simulink library "UoA_3D_LRd_2008"  (R2014b)
settings: Solver=ode45  StartTime=0.0  StopTime=10.0  RelTol=1e-3
libraries: simulink_extras x2, simulink x2
settings Model: Creator=eyip002-admin  LastModifiedBy=nall426

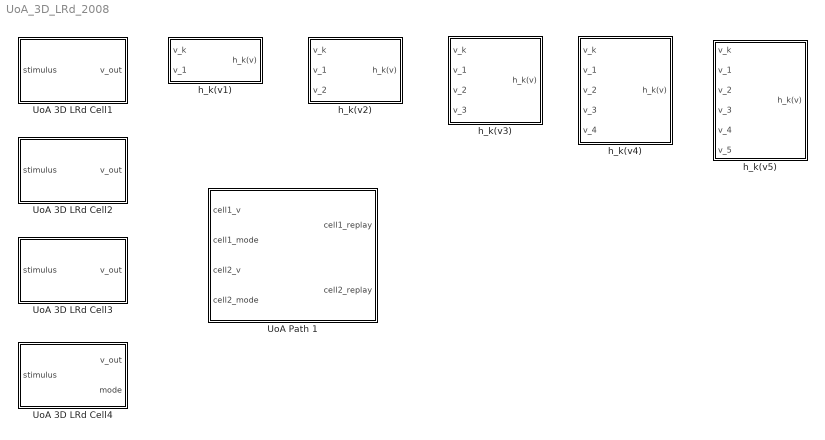
== system UoA_3D_LRd_2008 ==
  UoA 3D LRd Cell1 : Subsystem  mask{V_T=44.5, V_R=30, V_O_max=131.1, alpha0_x=-0.0087, alpha1_x=-0.0236, alpha2_x=-0.0069, alpha3_x=-0.0332, alpha0_y=-0.1909, alpha1_y=-0.0455, alpha2_y=0.0759, alpha3_y=0.0280, alpha0_z=-0.1904, alpha1_z=-0.0129, alpha2_z=6.8265, alpha3_z=0.0020, v_n_R_max=5e-9, v_n_R_min=3.04e-9, i_st_x=0, i_st_y=0, i_st_z=0, i_st_gx=0.7772, i_st_gy=0.0589, i_st_gz=0.2766}
      mask prompts: V_T "V_T (stimulation)"; V_R "V_R (resting)"; V_O_max "V_O_max (overshoot)"; v_n_R_max "v_n_R_max (Maximum rate)"; v_n_R_min "v_n_R_min (To correct transition error)"; i_st_x "i_st_x (x dimension)"; i_st_y "i_st_y (y dimension)"; i_st_z "i_st_z (z dimension)"
      mask DialogControl DescTextVar Prompt: Parameters for UoA 3D Luo-Rudy cardiac cell. Based on Stony Brook's 2008 3D HA LRd model with modifications.
      mask Display:
      | disp('Isolated_1\n(2008)')
      | port_label('input', 1, 'stim')
      | port_label('output', 1, 'v_k')
  UoA 3D LRd Cell2 : Subsystem  mask{V_T=44.5, V_R=30, V_O_max=131.1, alpha0_x=-0.0087, alpha1_x=-0.0236, alpha2_x=-0.0069, alpha3_x=-0.0332, alpha0_y=-0.1909, alpha1_y=-0.0455, alpha2_y=0.0759, alpha3_y=0.0280, alpha0_z=-0.1904, alpha1_z=-0.0129, alpha2_z=6.8265, alpha3_z=0.0020, v_n_R_max=5e-9, v_n_R_min=3.04e-9, i_st_x=0, i_st_y=0, i_st_z=0, i_st_gx=0.7772, i_st_gy=0.0589, i_st_gz=0.2766}
      mask prompts: V_T "V_T (stimulation)"; V_R "V_R (resting)"; V_O_max "V_O_max (overshoot)"; v_n_R_max "v_n_R_max (Maximum rate)"; v_n_R_min "v_n_R_min (To correct transition error)"; i_st_x "i_st_x (x dimension)"; i_st_y "i_st_y (y dimension)"; i_st_z "i_st_z (z dimension)"
      mask DialogControl DescTextVar Prompt: Parameters for UoA 3D Luo-Rudy cardiac cell. Based on Stony Brook's 2008 3D HA LRd model with modifications.
      mask Display:
      | disp('Isolated_2\n(2008)')
      | port_label('input', 1, 'stim')
      | port_label('output', 1, 'v_k')
  UoA 3D LRd Cell3 : Subsystem  mask{V_T=44.5, V_R=30, V_O_max=131.1, alpha0_x=-0.0087, alpha1_x=-0.0236, alpha2_x=-0.0069, alpha3_x=-0.0332, alpha0_y=-0.1909, alpha1_y=-0.0455, alpha2_y=0.0759, alpha3_y=0.0280, alpha0_z=-0.1904, alpha1_z=-0.0129, alpha2_z=6.8265, alpha3_z=0.0020, v_n_R_max=0.04, i_st_gx=0.7772, i_st_gy=0.0589, i_st_gz=0.2766}
      mask prompts: V_T "V_T (stimulation)"; V_R "V_R (resting)"; V_O_max "V_O_max (overshoot)"; v_n_R_max "v_n_R_max (Maximum rate)"
      mask DialogControl DescTextVar Prompt: Parameters for UoA 3D Luo-Rudy cardiac cell. Based on Stony Brook's 2008 3D HA LRd model with modifications.
      mask DialogControl Container10 Prompt: Stimulus current as a proportion of incoming voltages
      mask Display:
      | disp('Isolated_3\n(2008)')
      | port_label('input', 1, 'stim')
      | port_label('output', 1, 'v_k')
  UoA 3D LRd Cell4 : Subsystem  mask{V_T=44.5, V_R=30, V_O_max=131.1, alpha0_x=-0.0087, alpha1_x=-0.0236, alpha2_x=-0.0069, alpha3_x=-0.0332, alpha0_y=-0.1909, alpha1_y=-0.0455, alpha2_y=0.0759, alpha3_y=0.0280, alpha0_z=-0.1904, alpha1_z=-0.0129, alpha2_z=6.8265, alpha3_z=0.0020, v_n_R_max=0.04, i_st_gx=0.7772, i_st_gy=0.0589, i_st_gz=0.2766}
      mask prompts: V_T "V_T (stimulation)"; V_R "V_R (resting)"; V_O_max "V_O_max (overshoot)"; v_n_R_max "v_n_R_max (Maximum rate)"
      mask DialogControl DescTextVar Prompt: Parameters for UoA 3D Luo-Rudy cardiac cell. Based on Stony Brook's 3D HA LRd model with modifications.
      mask DialogControl Container10 Prompt: Stimulus current as a proportion of incoming voltages
      mask Display:
      | disp('Isolated_4\n(2008)')
      | port_label('input', 1, 'stim')
      | port_label('output', 1, 'v_k')
      | port_label('output', 2, 'mode')
  UoA Path 1 : Subsystem  mask{cell1_conduction_time=1, cell2_conduction_time=1, cell1_charge_time=1, cell2_charge_time=1}
      mask prompts: cell1_conduction_time "Cell 1 to cell 2"; cell2_conduction_time "Cell 2 to cell 1"; cell1_charge_time "Cell 1"; cell2_charge_time "Cell 2"
      mask DialogControl DescTextVar Prompt: Parameters for the UoA path model. Based on the UPenn path model with modifications.
      mask Display:
      | disp('UoA_1')
      | port_label('input', 1, 'cell1_v')
      | port_label('input', 2, 'cell1_mode')
      | port_label('input', 3, 'cell2_v')
      | port_label('input', 4, 'cell2_mode')
      | port_label('output', 1, 'cell1_replay')
      | port_label('output', 2, 'cell2_replay')
  h_k(v1) : Subsystem  mask{A_m=10*10, C_m=1/(10*10), G_1=10*10, s_1=1/10, d_1=10}
      mask prompts: A_m "A_m (Cell surface area to cell volume)"; C_m "C_m (Specific membrane capacitance)"
      mask DialogControl DescTextVar Prompt: University of Auckland's voltage aggregation function, h(v).
      mask Display:
      | disp('UoA_1')
      | port_label('input', 1, 'v_k')
      | port_label('input', 2, 'v_1')
      | port_label('output', 1, 'h_k')
  h_k(v2) : Subsystem  mask{A_m=10*10, C_m=1/(10*10), G_1=10*10, G_2=10*10, s_1=1/10, s_2=1/10, d_1=10, d_2=10}
      mask prompts: A_m "A_m (Cell surface area to cell volume)"; C_m "C_m (Specific membrane capacitance)"
      mask DialogControl DescTextVar Prompt: University of Auckland's voltage aggregation function, h(v).
      mask Display:
      | disp('UoA_1')
      | port_label('input', 1, 'v_k')
      | port_label('input', 2, 'v_1')
      | port_label('input', 3, 'v_2')
      | port_label('output', 1, 'h_k')
  h_k(v3) : Subsystem  mask{A_m=10*10, C_m=1/(10*10), G_1=10*10, G_2=10*10, G_3=10*10, s_1=1/10, s_2=1/10, s_3=1/10, d_1=10, d_2=10, d_3=10}
      mask prompts: A_m "A_m (Cell surface area to cell volume)"; C_m "C_m (Specific membrane capacitance)"
      mask DialogControl DescTextVar Prompt: University of Auckland's voltage aggregation function, h(v).
      mask Display:
      | disp('UoA_1')
      | port_label('input', 1, 'v_k')
      | port_label('input', 2, 'v_1')
      | port_label('input', 3, 'v_2')
      | port_label('input', 4, 'v_3')
      | port_label('output', 1, 'h_k')
  h_k(v4) : Subsystem  mask{A_m=10*10, C_m=1/(10*10), G_1=10*10, G_2=10*10, G_3=10*10, G_4=10*10, s_1=1/10, s_2=1/10, s_3=1/10, s_4=1/10, d_1=10, d_2=10, d_3=10, d_4=10}
      mask prompts: A_m "A_m (Cell surface area to cell volume)"; C_m "C_m (Specific membrane capacitance)"
      mask DialogControl DescTextVar Prompt: University of Auckland's voltage aggregation function, h(v).
      mask Display:
      | disp('UoA_1')
      | port_label('input', 1, 'v_k')
      | port_label('input', 2, 'v_1')
      | port_label('input', 3, 'v_2')
      | port_label('input', 4, 'v_3')
      | port_label('input', 5, 'v_4')
      | port_label('output', 1, 'h_k')
  h_k(v5) : Subsystem  mask{A_m=10*10, C_m=1/(10*10), G_1=10*10, G_2=10*10, G_3=10*10, G_4=10*10, G_5=10*10, s_1=1/10, s_2=1/10, s_3=1/10, s_4=1/10, s_5=1/10, d_1=10, d_2=10, d_3=10, d_4=10, d_5=10}
      mask prompts: A_m "A_m (Cell surface area to cell volume)"; C_m "C_m (Specific membrane capacitance)"
      mask DialogControl DescTextVar Prompt: University of Auckland's voltage aggregation function, h(v).
      mask Display:
      | disp('UoA_1')
      | port_label('input', 1, 'v_k')
      | port_label('input', 2, 'v_1')
      | port_label('input', 3, 'v_2')
      | port_label('input', 4, 'v_3')
      | port_label('input', 5, 'v_4')
      | port_label('input', 6, 'v_5')
      | port_label('output', 1, 'h_k')

== system UoA_3D_LRd_2008/UoA 3D LRd Cell1 ==
  stimulus : Inport
  Modes and Transitions : Stateflow chart  TreatAsAtomicUnit=on
  V_O_max : Constant  Value=V_O_max
  V_R : Constant  Value=V_R
  V_T : Constant  Value=V_T
  v_(x,y,z) Computation : Subsystem
  v_out : Outport
  wires:
  Modes and Transitions/2(v_n_R) -> v_(x,y,z) Computation/3(v_n_R)
  Modes and Transitions/1(Mode) -> v_(x,y,z) Computation/2(Mode)
  v_(x,y,z) Computation/2(v_x_next) -> Modes and Transitions/5(v_x)
  Modes and Transitions/3(v_x_reset) -> v_(x,y,z) Computation/4(v_x_reset)
  Modes and Transitions/6(reset) -> v_(x,y,z) Computation/7(reset)
  v_(x,y,z) Computation/3(v_y_next) -> Modes and Transitions/6(v_y)
  v_(x,y,z) Computation/4(v_z_next) -> Modes and Transitions/7(v_z)
  Modes and Transitions/4(v_y_reset) -> v_(x,y,z) Computation/5(v_y_reset)
  Modes and Transitions/5(v_z_reset) -> v_(x,y,z) Computation/6(v_z_reset)
  stimulus/1 -> v_(x,y,z) Computation/1(g(v)), Modes and Transitions/1(stimulus)
  v_(x,y,z) Computation/1(v_out) -> v_out/1
  V_T/1 -> Modes and Transitions/2(V_T)
  V_R/1 -> Modes and Transitions/3(V_R)
  V_O_max/1 -> Modes and Transitions/4(V_O_max)

== system UoA_3D_LRd_2008/UoA 3D LRd Cell2 ==
  stimulus : Inport
  Modes and Transitions : Stateflow chart  TreatAsAtomicUnit=on
  V_O_max : Constant  Value=V_O_max
  V_R : Constant  Value=V_R
  V_T : Constant  Value=V_T
  v_(x,y,z) Computation : Subsystem
  v_out : Outport
  wires:
  Modes and Transitions/2(v_n_R) -> v_(x,y,z) Computation/3(v_n_R)
  Modes and Transitions/1(Mode) -> v_(x,y,z) Computation/2(Mode)
  v_(x,y,z) Computation/2(v_x_next) -> Modes and Transitions/5(v_x)
  Modes and Transitions/3(v_x_reset) -> v_(x,y,z) Computation/4(v_x_reset)
  Modes and Transitions/6(reset) -> v_(x,y,z) Computation/7(reset)
  v_(x,y,z) Computation/3(v_y_next) -> Modes and Transitions/6(v_y)
  v_(x,y,z) Computation/4(v_z_next) -> Modes and Transitions/7(v_z)
  Modes and Transitions/4(v_y_reset) -> v_(x,y,z) Computation/5(v_y_reset)
  Modes and Transitions/5(v_z_reset) -> v_(x,y,z) Computation/6(v_z_reset)
  stimulus/1 -> v_(x,y,z) Computation/1(g(v)), Modes and Transitions/1(stimulus)
  v_(x,y,z) Computation/1(v_out) -> v_out/1
  V_T/1 -> Modes and Transitions/2(V_T)
  V_R/1 -> Modes and Transitions/3(V_R)
  V_O_max/1 -> Modes and Transitions/4(V_O_max)

== system UoA_3D_LRd_2008/UoA 3D LRd Cell3 ==
  stimulus : Inport
  Modes and Transitions : Stateflow chart  TreatAsAtomicUnit=on
  V_O_max : Constant  Value=V_O_max
  V_R : Constant  Value=V_R
  V_T : Constant  Value=V_T
  v_(x,y,z) Computation : Subsystem
  v_out : Outport
  wires:
  Modes and Transitions/2(v_n_R) -> v_(x,y,z) Computation/3(v_n_R)
  Modes and Transitions/1(Mode) -> v_(x,y,z) Computation/2(Mode)
  v_(x,y,z) Computation/2(v_x_next) -> Modes and Transitions/5(v_x)
  Modes and Transitions/3(v_x_reset) -> v_(x,y,z) Computation/4(v_x_reset)
  Modes and Transitions/6(reset) -> v_(x,y,z) Computation/7(reset)
  v_(x,y,z) Computation/3(v_y_next) -> Modes and Transitions/6(v_y)
  v_(x,y,z) Computation/4(v_z_next) -> Modes and Transitions/7(v_z)
  Modes and Transitions/4(v_y_reset) -> v_(x,y,z) Computation/5(v_y_reset)
  Modes and Transitions/5(v_z_reset) -> v_(x,y,z) Computation/6(v_z_reset)
  stimulus/1 -> v_(x,y,z) Computation/1(g(v)), Modes and Transitions/1(stimulus)
  v_(x,y,z) Computation/1(v_out) -> v_out/1
  V_T/1 -> Modes and Transitions/2(V_T)
  V_R/1 -> Modes and Transitions/3(V_R)
  V_O_max/1 -> Modes and Transitions/4(V_O_max)

== system UoA_3D_LRd_2008/UoA 3D LRd Cell4 ==
  stimulus : Inport
  Modes and Transitions : Stateflow chart  TreatAsAtomicUnit=on
  V_O_max : Constant  Value=V_O_max
  V_R : Constant  Value=V_R
  V_T : Constant  Value=V_T
  v_(x,y,z) Computation : Subsystem
  v_out : Outport
  mode : Outport  Port=2
  wires:
  V_O_max/1 -> Modes and Transitions/4(V_O_max)
  V_R/1 -> Modes and Transitions/3(V_R)
  V_T/1 -> Modes and Transitions/2(V_T)
  v_(x,y,z) Computation/1(v_out) -> v_out/1
  stimulus/1 -> Modes and Transitions/1(stimulus), v_(x,y,z) Computation/1(g(v))
  Modes and Transitions/5(v_z_reset) -> v_(x,y,z) Computation/6(v_z_reset)
  Modes and Transitions/4(v_y_reset) -> v_(x,y,z) Computation/5(v_y_reset)
  v_(x,y,z) Computation/4(v_z_next) -> Modes and Transitions/7(v_z)
  v_(x,y,z) Computation/3(v_y_next) -> Modes and Transitions/6(v_y)
  Modes and Transitions/6(reset) -> v_(x,y,z) Computation/7(reset)
  Modes and Transitions/3(v_x_reset) -> v_(x,y,z) Computation/4(v_x_reset)
  v_(x,y,z) Computation/2(v_x_next) -> Modes and Transitions/5(v_x)
  Modes and Transitions/1(Mode) -> mode/1, v_(x,y,z) Computation/2(Mode)
  Modes and Transitions/2(v_n_R) -> v_(x,y,z) Computation/3(v_n_R)

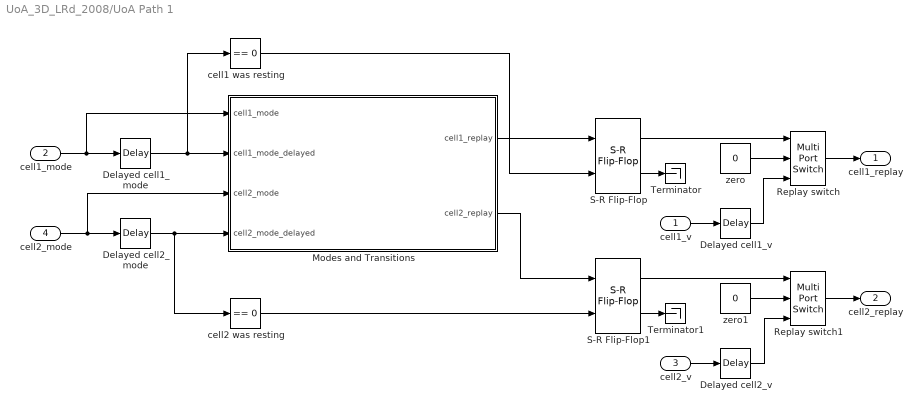
== system UoA_3D_LRd_2008/UoA Path 1 ==
  cell1_v : Inport
  cell1_mode : Inport  Port=2
  cell2_v : Inport  Port=3
  cell2_mode : Inport  Port=4
  Delayed cell1_mode : TransportDelay  DelayTime=cell1_conduction_time  BufferSize=200704
  Delayed cell1_v : TransportDelay  DelayTime=cell1_conduction_time  BufferSize=200704
  Delayed cell2_mode : TransportDelay  DelayTime=cell2_conduction_time  BufferSize=200704
  Delayed cell2_v : TransportDelay  DelayTime=cell2_conduction_time  BufferSize=200704
  Modes and Transitions : Stateflow chart  TreatAsAtomicUnit=on
  Replay switch : MultiPortSwitch  DataPortOrder=Zero-based contiguous  Inputs=2
  Replay switch1 : MultiPortSwitch  DataPortOrder=Zero-based contiguous  Inputs=2
  S-R Flip-Flop : simulink_extras/Flip Flops/S-R Flip-Flop  initial_condition=0
  S-R Flip-Flop1 : simulink_extras/Flip Flops/S-R Flip-Flop  initial_condition=0
  Terminator : Terminator
  Terminator1 : Terminator
  cell1 was resting : simulink/Logic and Bit Operations/Compare To Constant  relop===  const=0  OutDataTypeStr=boolean
  cell2 was resting : simulink/Logic and Bit Operations/Compare To Constant  relop===  const=0  OutDataTypeStr=boolean
  zero : Constant  Value=0
  zero1 : Constant  Value=0
  cell1_replay : Outport
  cell2_replay : Outport  Port=2
  wires:
  cell2_mode/1 -> Modes and Transitions/3(cell2_mode), Delayed cell2_mode/1
  cell1_mode/1 -> Modes and Transitions/1(cell1_mode), Delayed cell1_mode/1
  Replay switch/1 -> cell1_replay/1
  Replay switch1/1 -> cell2_replay/1
  zero/1 -> Replay switch/2
  zero1/1 -> Replay switch1/2
  cell2_v/1 -> Delayed cell2_v/1
  cell1_v/1 -> Delayed cell1_v/1
  Delayed cell2_v/1 -> Replay switch1/3
  Delayed cell1_v/1 -> Replay switch/3
  Delayed cell2_mode/1 -> Modes and Transitions/4(cell2_mode_delayed), cell2 was resting/1
  Delayed cell1_mode/1 -> cell1 was resting/1, Modes and Transitions/2(cell1_mode_delayed)
  S-R Flip-Flop1/1 -> Replay switch1/1
  S-R Flip-Flop1/2 -> Terminator1/1
  S-R Flip-Flop/2 -> Terminator/1
  S-R Flip-Flop/1 -> Replay switch/1
  Modes and Transitions/2(cell2_replay) -> S-R Flip-Flop1/1
  Modes and Transitions/1(cell1_replay) -> S-R Flip-Flop/1
  cell1 was resting/1 -> S-R Flip-Flop/2
  cell2 was resting/1 -> S-R Flip-Flop1/2

== system UoA_3D_LRd_2008/h_k(v1) ==
  v_k : Inport
  v_1 : Inport  Port=2
  Diffusion_1 : Constant  Value=(G_1*s_1)/(A_m*C_m*d_1)
  Product : Product
  Subtract : Sum  Inputs=+-
  h_k(v) : Outport
  wires:
  Product/1 -> h_k(v)/1
  v_k/1 -> Subtract/2
  v_1/1 -> Subtract/1
  Subtract/1 -> Product/2
  Diffusion_1/1 -> Product/1

== system UoA_3D_LRd_2008/h_k(v2) ==
  v_k : Inport
  v_1 : Inport  Port=2
  v_2 : Inport  Port=3
  Diffusion_1 : Constant  Value=(G_1*s_1)/(A_m*C_m*d_1)
  Diffusion_2 : Constant  Value=(G_2*s_2)/(A_m*C_m*d_2)
  Product : Product
  Product1 : Product
  Subtract : Sum  Inputs=+-
  Subtract1 : Sum  Inputs=+-
  Sum : Sum
  h_k(v) : Outport
  wires:
  Sum/1 -> h_k(v)/1
  v_k/1 -> Subtract/2, Subtract1/2
  v_1/1 -> Subtract/1
  Subtract/1 -> Product/2
  Diffusion_1/1 -> Product/1
  Product/1 -> Sum/1
  v_2/1 -> Subtract1/1
  Subtract1/1 -> Product1/2
  Diffusion_2/1 -> Product1/1
  Product1/1 -> Sum/2

== system UoA_3D_LRd_2008/h_k(v3) ==
  v_k : Inport
  v_1 : Inport  Port=2
  v_2 : Inport  Port=3
  v_3 : Inport  Port=4
  Diffusion_1 : Constant  Value=(G_1*s_1)/(A_m*C_m*d_1)
  Diffusion_2 : Constant  Value=(G_2*s_2)/(A_m*C_m*d_2)
  Diffusion_3 : Constant  Value=(G_3*s_3)/(A_m*C_m*d_3)
  Product : Product
  Product1 : Product
  Product2 : Product
  Subtract : Sum  Inputs=+-
  Subtract1 : Sum  Inputs=+-
  Subtract2 : Sum  Inputs=+-
  Sum : Sum  Inputs=+++
  h_k(v) : Outport
  wires:
  Sum/1 -> h_k(v)/1
  v_1/1 -> Subtract/1
  Subtract/1 -> Product/2
  Diffusion_1/1 -> Product/1
  Product/1 -> Sum/1
  v_2/1 -> Subtract1/1
  Subtract1/1 -> Product1/2
  Diffusion_2/1 -> Product1/1
  Product1/1 -> Sum/2
  v_k/1 -> Subtract/2, Subtract1/2, Subtract2/2
  v_3/1 -> Subtract2/1
  Subtract2/1 -> Product2/2
  Diffusion_3/1 -> Product2/1
  Product2/1 -> Sum/3

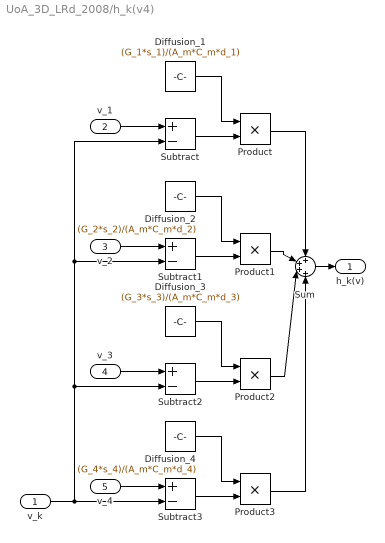
== system UoA_3D_LRd_2008/h_k(v4) ==
  v_k : Inport
  v_1 : Inport  Port=2
  v_2 : Inport  Port=3
  v_3 : Inport  Port=4
  v_4 : Inport  Port=5
  Diffusion_1 : Constant  Value=(G_1*s_1)/(A_m*C_m*d_1)
  Diffusion_2 : Constant  Value=(G_2*s_2)/(A_m*C_m*d_2)
  Diffusion_3 : Constant  Value=(G_3*s_3)/(A_m*C_m*d_3)
  Diffusion_4 : Constant  Value=(G_4*s_4)/(A_m*C_m*d_4)
  Product{,1..3} (4 alike) : Product
  Subtract{,1..3} (4 alike) : Sum  Inputs=+-
  Sum : Sum  Inputs=++++
  h_k(v) : Outport
  wires:
  Sum/1 -> h_k(v)/1
  v_1/1 -> Subtract/1
  Subtract/1 -> Product/2
  Diffusion_1/1 -> Product/1
  Product/1 -> Sum/1
  v_2/1 -> Subtract1/1
  Subtract1/1 -> Product1/2
  Diffusion_2/1 -> Product1/1
  Product1/1 -> Sum/2
  v_3/1 -> Subtract2/1
  Subtract2/1 -> Product2/2
  Diffusion_3/1 -> Product2/1
  Product2/1 -> Sum/3
  v_k/1 -> Subtract/2, Subtract1/2, Subtract2/2, Subtract3/2
  v_4/1 -> Subtract3/1
  Subtract3/1 -> Product3/2
  Diffusion_4/1 -> Product3/1
  Product3/1 -> Sum/4

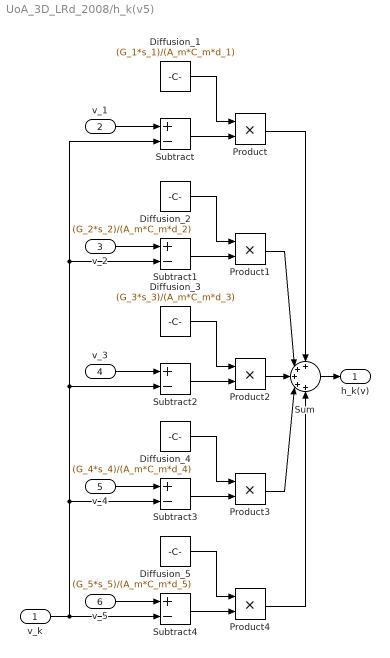
== system UoA_3D_LRd_2008/h_k(v5) ==
  v_k : Inport
  v_1 : Inport  Port=2
  v_2 : Inport  Port=3
  v_3 : Inport  Port=4
  v_4 : Inport  Port=5
  v_5 : Inport  Port=6
  Diffusion_1 : Constant  Value=(G_1*s_1)/(A_m*C_m*d_1)
  Diffusion_2 : Constant  Value=(G_2*s_2)/(A_m*C_m*d_2)
  Diffusion_3 : Constant  Value=(G_3*s_3)/(A_m*C_m*d_3)
  Diffusion_4 : Constant  Value=(G_4*s_4)/(A_m*C_m*d_4)
  Diffusion_5 : Constant  Value=(G_5*s_5)/(A_m*C_m*d_5)
  Product{,1..4} (5 alike) : Product
  Subtract{,1..4} (5 alike) : Sum  Inputs=+-
  Sum : Sum  Inputs=+++++
  h_k(v) : Outport
  wires:
  Sum/1 -> h_k(v)/1
  v_1/1 -> Subtract/1
  Subtract/1 -> Product/2
  Diffusion_1/1 -> Product/1
  Product/1 -> Sum/1
  v_2/1 -> Subtract1/1
  Subtract1/1 -> Product1/2
  Diffusion_2/1 -> Product1/1
  Product1/1 -> Sum/2
  v_3/1 -> Subtract2/1
  Subtract2/1 -> Product2/2
  Diffusion_3/1 -> Product2/1
  Product2/1 -> Sum/3
  v_4/1 -> Subtract3/1
  Subtract3/1 -> Product3/2
  Diffusion_4/1 -> Product3/1
  Product3/1 -> Sum/4
  v_k/1 -> Subtract4/2, Subtract/2, Subtract1/2, Subtract2/2, Subtract3/2
  v_5/1 -> Subtract4/1
  Subtract4/1 -> Product4/2
  Diffusion_5/1 -> Product4/1
  Product4/1 -> Sum/5

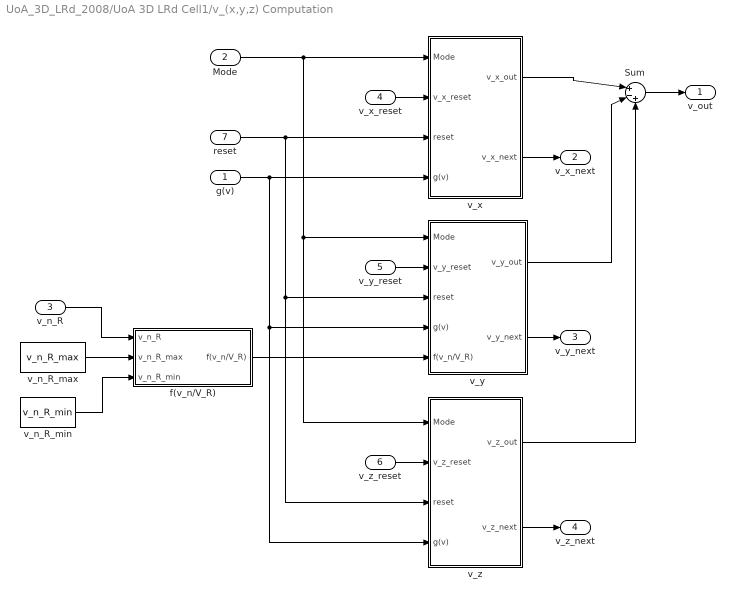
== system UoA_3D_LRd_2008/UoA 3D LRd Cell1/v_(x,y,z) Computation ==
  g(v) : Inport
  Mode : Inport  Port=2
  v_n_R : Inport  Port=3
  v_x_reset : Inport  Port=4
  v_y_reset : Inport  Port=5
  v_z_reset : Inport  Port=6
  reset : Inport  Port=7
  Sum : Sum  Inputs=|+-+
  f(v_n/V_R) : Subsystem
  v_n_R_max : Constant  Value=v_n_R_max
  v_n_R_min : Constant  Value=v_n_R_min
  v_x : Subsystem
  v_y : Subsystem
  v_z : Subsystem
  v_out : Outport
  v_x_next : Outport  Port=2
  v_y_next : Outport  Port=3
  v_z_next : Outport  Port=4
  wires:
  v_x_reset/1 -> v_x/2(v_x_reset)
  v_x/2(v_x_next) -> v_x_next/1
  v_y/2(v_y_next) -> v_y_next/1
  Mode/1 -> v_z/1(Mode), v_y/1(Mode), v_x/1(Mode)
  v_z/2(v_z_next) -> v_z_next/1
  Sum/1 -> v_out/1
  v_x/1(v_x_out) -> Sum/1
  v_y/1(v_y_out) -> Sum/2
  v_z/1(v_z_out) -> Sum/3
  v_y_reset/1 -> v_y/2(v_y_reset)
  v_z_reset/1 -> v_z/2(v_z_reset)
  g(v)/1 -> v_x/4(g(v)), v_z/4(g(v)), v_y/4(g(v))
  reset/1 -> v_z/3(reset), v_y/3(reset), v_x/3(reset)
  v_n_R_max/1 -> f(v_n/V_R)/2(v_n_R_max)
  v_n_R/1 -> f(v_n/V_R)/1(v_n_R)
  f(v_n/V_R)/1(f(v_n/V_R)) -> v_y/5(f(v_n/V_R))
  v_n_R_min/1 -> f(v_n/V_R)/3(v_n_R_min)

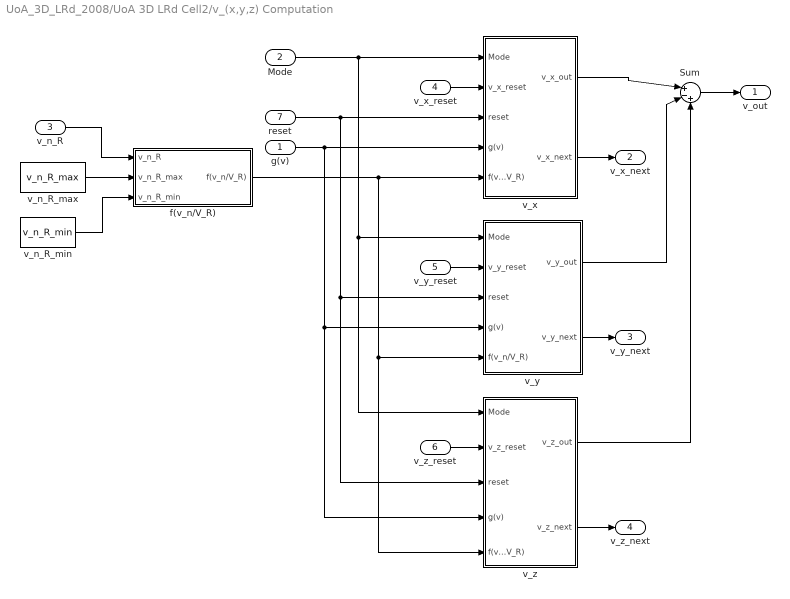
== system UoA_3D_LRd_2008/UoA 3D LRd Cell2/v_(x,y,z) Computation ==
  g(v) : Inport
  Mode : Inport  Port=2
  v_n_R : Inport  Port=3
  v_x_reset : Inport  Port=4
  v_y_reset : Inport  Port=5
  v_z_reset : Inport  Port=6
  reset : Inport  Port=7
  Sum : Sum  Inputs=|+-+
  f(v_n/V_R) : Subsystem
  v_n_R_max : Constant  Value=v_n_R_max
  v_n_R_min : Constant  Value=v_n_R_min
  v_x : Subsystem
  v_y : Subsystem
  v_z : Subsystem
  v_out : Outport
  v_x_next : Outport  Port=2
  v_y_next : Outport  Port=3
  v_z_next : Outport  Port=4
  wires:
  v_x_reset/1 -> v_x/2(v_x_reset)
  v_x/2(v_x_next) -> v_x_next/1
  v_y/2(v_y_next) -> v_y_next/1
  Mode/1 -> v_z/1(Mode), v_y/1(Mode), v_x/1(Mode)
  v_z/2(v_z_next) -> v_z_next/1
  Sum/1 -> v_out/1
  v_x/1(v_x_out) -> Sum/1
  v_y/1(v_y_out) -> Sum/2
  v_z/1(v_z_out) -> Sum/3
  v_y_reset/1 -> v_y/2(v_y_reset)
  v_z_reset/1 -> v_z/2(v_z_reset)
  g(v)/1 -> v_z/4(g(v)), v_y/4(g(v)), v_x/4(g(v))
  reset/1 -> v_z/3(reset), v_y/3(reset), v_x/3(reset)
  v_n_R_max/1 -> f(v_n/V_R)/2(v_n_R_max)
  v_n_R/1 -> f(v_n/V_R)/1(v_n_R)
  f(v_n/V_R)/1(f(v_n/V_R)) -> v_z/5(f(v_n/V_R)), v_y/5(f(v_n/V_R)), v_x/5(f(v_n/V_R))
  v_n_R_min/1 -> f(v_n/V_R)/3(v_n_R_min)

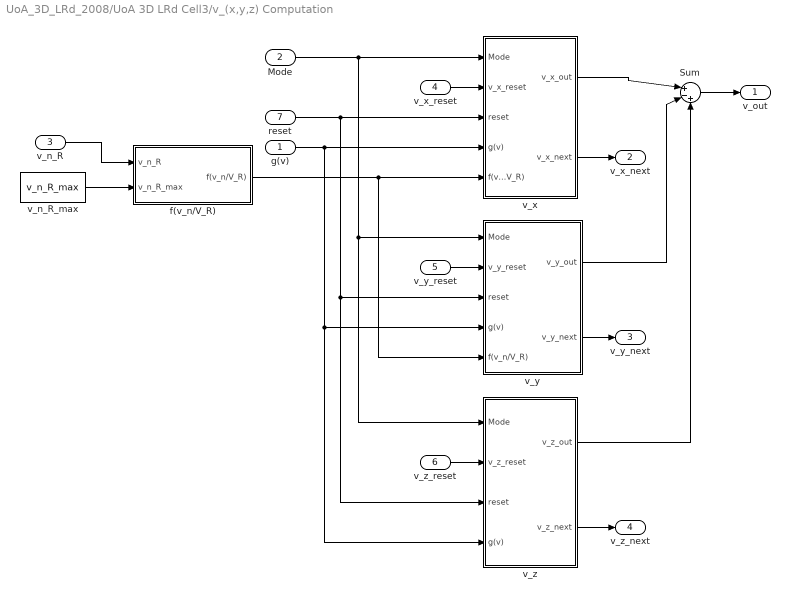
== system UoA_3D_LRd_2008/UoA 3D LRd Cell3/v_(x,y,z) Computation ==
  g(v) : Inport
  Mode : Inport  Port=2
  v_n_R : Inport  Port=3
  v_x_reset : Inport  Port=4
  v_y_reset : Inport  Port=5
  v_z_reset : Inport  Port=6
  reset : Inport  Port=7
  Sum : Sum  Inputs=|+-+
  f(v_n/V_R) : Subsystem
  v_n_R_max : Constant  Value=v_n_R_max
  v_x : Subsystem
  v_y : Subsystem
  v_z : Subsystem
  v_out : Outport
  v_x_next : Outport  Port=2
  v_y_next : Outport  Port=3
  v_z_next : Outport  Port=4
  wires:
  v_x_reset/1 -> v_x/2(v_x_reset)
  v_x/2(v_x_next) -> v_x_next/1
  v_y/2(v_y_next) -> v_y_next/1
  Mode/1 -> v_z/1(Mode), v_y/1(Mode), v_x/1(Mode)
  v_z/2(v_z_next) -> v_z_next/1
  Sum/1 -> v_out/1
  v_x/1(v_x_out) -> Sum/1
  v_y/1(v_y_out) -> Sum/2
  v_z/1(v_z_out) -> Sum/3
  v_y_reset/1 -> v_y/2(v_y_reset)
  v_z_reset/1 -> v_z/2(v_z_reset)
  g(v)/1 -> v_z/4(g(v)), v_y/4(g(v)), v_x/4(g(v))
  reset/1 -> v_z/3(reset), v_y/3(reset), v_x/3(reset)
  v_n_R_max/1 -> f(v_n/V_R)/2(v_n_R_max)
  v_n_R/1 -> f(v_n/V_R)/1(v_n_R)
  f(v_n/V_R)/1(f(v_n/V_R)) -> v_y/5(f(v_n/V_R)), v_x/5(f(v_n/V_R))

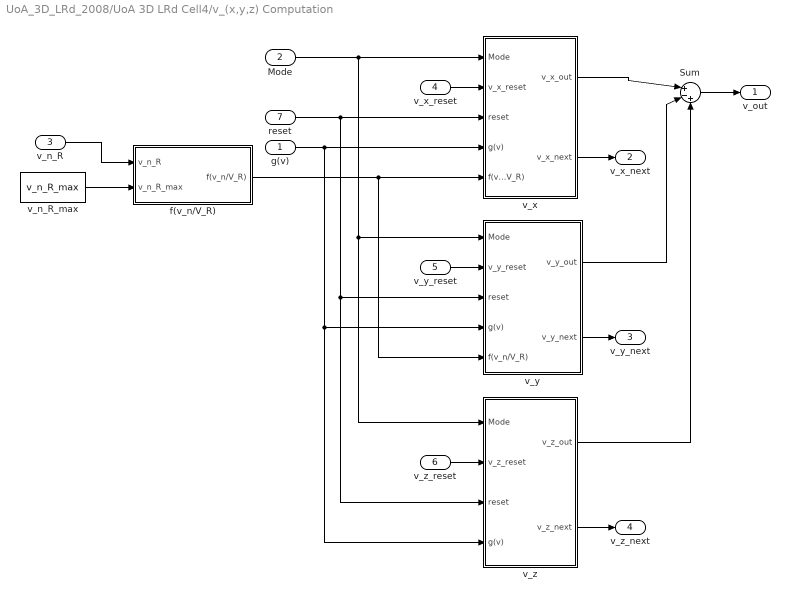
== system UoA_3D_LRd_2008/UoA 3D LRd Cell4/v_(x,y,z) Computation ==
  g(v) : Inport
  Mode : Inport  Port=2
  v_n_R : Inport  Port=3
  v_x_reset : Inport  Port=4
  v_y_reset : Inport  Port=5
  v_z_reset : Inport  Port=6
  reset : Inport  Port=7
  Sum : Sum  Inputs=|+-+
  f(v_n/V_R) : Subsystem
  v_n_R_max : Constant  Value=v_n_R_max
  v_x : Subsystem
  v_y : Subsystem
  v_z : Subsystem
  v_out : Outport
  v_x_next : Outport  Port=2
  v_y_next : Outport  Port=3
  v_z_next : Outport  Port=4
  wires:
  f(v_n/V_R)/1(f(v_n/V_R)) -> v_x/5(f(v_n/V_R)), v_y/5(f(v_n/V_R))
  v_n_R/1 -> f(v_n/V_R)/1(v_n_R)
  v_n_R_max/1 -> f(v_n/V_R)/2(v_n_R_max)
  reset/1 -> v_x/3(reset), v_y/3(reset), v_z/3(reset)
  g(v)/1 -> v_x/4(g(v)), v_y/4(g(v)), v_z/4(g(v))
  v_z_reset/1 -> v_z/2(v_z_reset)
  v_y_reset/1 -> v_y/2(v_y_reset)
  v_z/1(v_z_out) -> Sum/3
  v_y/1(v_y_out) -> Sum/2
  v_x/1(v_x_out) -> Sum/1
  Sum/1 -> v_out/1
  Mode/1 -> v_x/1(Mode), v_y/1(Mode), v_z/1(Mode)
  v_x_reset/1 -> v_x/2(v_x_reset)
  v_z/2(v_z_next) -> v_z_next/1
  v_y/2(v_y_next) -> v_y_next/1
  v_x/2(v_x_next) -> v_x_next/1

== system UoA_3D_LRd_2008/UoA 3D LRd Cell1/v_(x,y,z) Computation/f(v_n//V_R) ==
  v_n_R : Inport
  v_n_R_max : Inport  Port=2
  v_n_R_min : Inport  Port=3
  -10.99 : Gain  Gain=-10.99
  0.29 : Gain  Gain=0.29
  0.70 : Gain  Gain=0.70
  62.89 : Gain  Gain=62.89
  Subtract : Sum  Inputs=-+
  Subtract1 : Sum  Inputs=+-
  Sum3 : Sum  Inputs=|++
  Switch : Switch  Criteria=u2 > Threshold
  Switch1 : Switch  Criteria=u2 > Threshold
  Zero : Constant  Value=0
  exp : Math  SaturateOnIntegerOverflow=on
  exp1 : Math  SaturateOnIntegerOverflow=on
  f(v_n/V_R) : Outport
  wires:
  Sum3/1 -> f(v_n/V_R)/1
  v_n_R_max/1 -> Switch/3, Subtract/2
  Switch1/1 -> Switch/1, Subtract/1
  Subtract/1 -> Switch/2
  ? -> Switch1/3, Subtract1/2
  v_n_R_min/1 -> Subtract1/1
  Subtract1/1 -> Switch1/2
  Zero/1 -> Switch1/1
  62.89/1 -> exp/1
  exp/1 -> 0.29/1
  -10.99/1 -> exp1/1
  exp1/1 -> 0.70/1
  0.29/1 -> Sum3/1
  0.70/1 -> Sum3/2
  v_n_R/1 -> 62.89/1, -10.99/1

== system UoA_3D_LRd_2008/UoA 3D LRd Cell1/v_(x,y,z) Computation/v_x ==
  Mode : Inport
  v_x_reset : Inport  Port=2
  reset : Inport  Port=3
  g(v) : Inport  Port=4
  Gain : Gain  Gain=i_st_gx
  Initial Condition : InitialCondition  Value=0
  Integrator : Integrator  ExternalReset=either  InitialConditionSource=external  ShowStatePort=on
  Multiport Switch : MultiPortSwitch  Inputs=4
  Sum1 : Sum  Inputs=++|
  alpha0 : Gain  Gain=alpha0_x
  alpha1 : Gain  Gain=alpha1_x
  alpha2 : Gain  Gain=alpha2_x
  alpha3 : Gain  Gain=alpha3_x
  v_x_out : Outport
  v_x_next : Outport  Port=2
  wires:
  alpha0/1 -> Multiport Switch/2
  alpha3/1 -> Multiport Switch/5
  alpha2/1 -> Multiport Switch/4
  Multiport Switch/1 -> Integrator/1
  Mode/1 -> Multiport Switch/1
  Gain/1 -> Sum1/1
  Integrator/1 -> alpha3/1, alpha1/1, alpha0/1, alpha2/1, v_x_out/1  "v_x"
  reset/1 -> Integrator/2
  v_x_reset/1 -> Initial Condition/1
  g(v)/1 -> Gain/1
  Initial Condition/1 -> Integrator/3
  Integrator/State -> v_x_next/1
  alpha1/1 -> Sum1/2
  Sum1/1 -> Multiport Switch/3

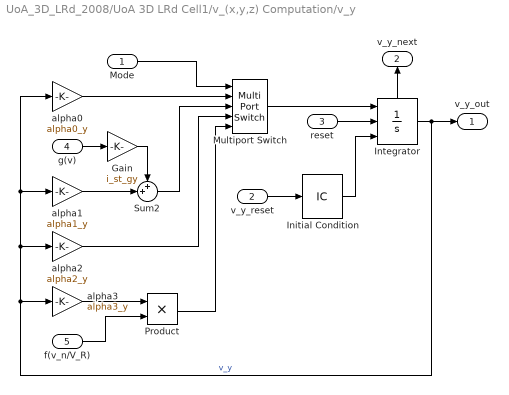
== system UoA_3D_LRd_2008/UoA 3D LRd Cell1/v_(x,y,z) Computation/v_y ==
  Mode : Inport
  v_y_reset : Inport  Port=2
  reset : Inport  Port=3
  g(v) : Inport  Port=4
  f(v_n/V_R) : Inport  Port=5
  Gain : Gain  Gain=i_st_gy
  Initial Condition : InitialCondition  Value=0
  Integrator : Integrator  ExternalReset=either  InitialConditionSource=external  ShowStatePort=on
  Multiport Switch : MultiPortSwitch  Inputs=4
  Product : Product  RndMeth=Zero
  Sum2 : Sum  Inputs=++|
  alpha0 : Gain  Gain=alpha0_y
  alpha1 : Gain  Gain=alpha1_y
  alpha2 : Gain  Gain=alpha2_y
  alpha3 : Gain  Gain=alpha3_y
  v_y_out : Outport
  v_y_next : Outport  Port=2
  wires:
  Integrator/1 -> v_y_out/1, alpha1/1, alpha0/1, alpha2/1, alpha3/1  "v_y"
  alpha2/1 -> Multiport Switch/4
  Multiport Switch/1 -> Integrator/1
  Mode/1 -> Multiport Switch/1
  Integrator/State -> v_y_next/1
  reset/1 -> Integrator/2
  v_y_reset/1 -> Initial Condition/1
  Initial Condition/1 -> Integrator/3
  Gain/1 -> Sum2/1
  g(v)/1 -> Gain/1
  alpha0/1 -> Multiport Switch/2
  f(v_n/V_R)/1 -> Product/2
  alpha3/1 -> Product/1
  Product/1 -> Multiport Switch/5
  alpha1/1 -> Sum2/2
  Sum2/1 -> Multiport Switch/3

== system UoA_3D_LRd_2008/UoA 3D LRd Cell1/v_(x,y,z) Computation/v_z ==
  Mode : Inport
  v_z_reset : Inport  Port=2
  reset : Inport  Port=3
  g(v) : Inport  Port=4
  Gain : Gain  Gain=i_st_gz
  Initial Condition : InitialCondition  Value=0
  Integrator : Integrator  ExternalReset=either  InitialConditionSource=external  ShowStatePort=on
  Multiport Switch : MultiPortSwitch  Inputs=4
  Sum2 : Sum  Inputs=++|
  alpha0 : Gain  Gain=alpha0_z
  alpha1 : Gain  Gain=alpha1_z
  alpha2 : Gain  Gain=alpha2_z
  alpha3 : Gain  Gain=alpha3_z
  v_z_out : Outport
  v_z_next : Outport  Port=2
  wires:
  Integrator/1 -> v_z_out/1, alpha1/1, alpha0/1, alpha2/1, alpha3/1  "v_z"
  alpha2/1 -> Multiport Switch/4
  Multiport Switch/1 -> Integrator/1
  Mode/1 -> Multiport Switch/1
  Integrator/State -> v_z_next/1
  reset/1 -> Integrator/2
  v_z_reset/1 -> Initial Condition/1
  Initial Condition/1 -> Integrator/3
  g(v)/1 -> Gain/1
  Gain/1 -> Sum2/1
  alpha0/1 -> Multiport Switch/2
  alpha3/1 -> Multiport Switch/5
  alpha1/1 -> Sum2/2
  Sum2/1 -> Multiport Switch/3

== system UoA_3D_LRd_2008/UoA 3D LRd Cell2/v_(x,y,z) Computation/f(v_n//V_R) ==
  v_n_R : Inport
  v_n_R_max : Inport  Port=2
  v_n_R_min : Inport  Port=3
  -10.99 : Gain  Gain=-10.99
  0.29 : Gain  Gain=0.29
  0.70 : Gain  Gain=0.70
  62.89 : Gain  Gain=62.89
  Subtract : Sum  Inputs=-+
  Subtract1 : Sum  Inputs=+-
  Sum3 : Sum  Inputs=|++
  Switch : Switch  Criteria=u2 > Threshold
  Switch1 : Switch  Criteria=u2 > Threshold
  Zero : Constant  Value=0
  exp : Math  SaturateOnIntegerOverflow=on
  exp1 : Math  SaturateOnIntegerOverflow=on
  f(v_n/V_R) : Outport
  wires:
  Sum3/1 -> f(v_n/V_R)/1
  v_n_R_max/1 -> Switch/3, Subtract/2
  Switch1/1 -> Switch/1, Subtract/1
  Subtract/1 -> Switch/2
  ? -> Switch1/3, Subtract1/2
  v_n_R_min/1 -> Subtract1/1
  Subtract1/1 -> Switch1/2
  Zero/1 -> Switch1/1
  62.89/1 -> exp/1
  exp/1 -> 0.29/1
  -10.99/1 -> exp1/1
  exp1/1 -> 0.70/1
  0.29/1 -> Sum3/1
  0.70/1 -> Sum3/2
  v_n_R/1 -> 62.89/1, -10.99/1

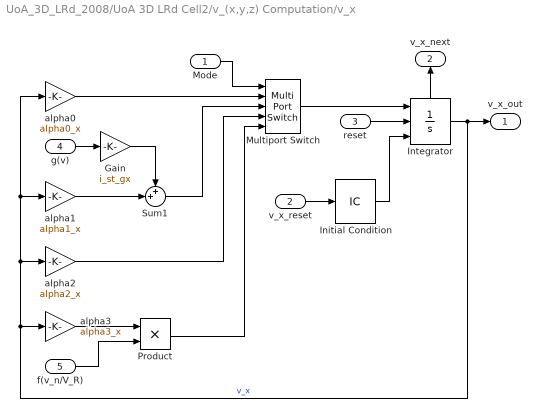
== system UoA_3D_LRd_2008/UoA 3D LRd Cell2/v_(x,y,z) Computation/v_x ==
  Mode : Inport
  v_x_reset : Inport  Port=2
  reset : Inport  Port=3
  g(v) : Inport  Port=4
  f(v_n/V_R) : Inport  Port=5
  Gain : Gain  Gain=i_st_gx
  Initial Condition : InitialCondition  Value=0
  Integrator : Integrator  ExternalReset=either  InitialConditionSource=external  ShowStatePort=on
  Multiport Switch : MultiPortSwitch  Inputs=4
  Product : Product  RndMeth=Zero
  Sum1 : Sum  Inputs=++|
  alpha0 : Gain  Gain=alpha0_x
  alpha1 : Gain  Gain=alpha1_x
  alpha2 : Gain  Gain=alpha2_x
  alpha3 : Gain  Gain=alpha3_x
  v_x_out : Outport
  v_x_next : Outport  Port=2
  wires:
  alpha0/1 -> Multiport Switch/2
  alpha2/1 -> Multiport Switch/4
  Multiport Switch/1 -> Integrator/1
  Mode/1 -> Multiport Switch/1
  Gain/1 -> Sum1/1
  Integrator/1 -> alpha3/1, alpha1/1, alpha0/1, alpha2/1, v_x_out/1  "v_x"
  reset/1 -> Integrator/2
  v_x_reset/1 -> Initial Condition/1
  g(v)/1 -> Gain/1
  Initial Condition/1 -> Integrator/3
  Integrator/State -> v_x_next/1
  alpha1/1 -> Sum1/2
  Sum1/1 -> Multiport Switch/3
  f(v_n/V_R)/1 -> Product/2
  alpha3/1 -> Product/1
  Product/1 -> Multiport Switch/5

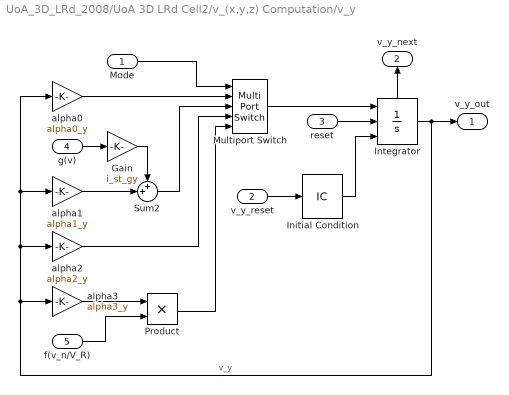
== system UoA_3D_LRd_2008/UoA 3D LRd Cell2/v_(x,y,z) Computation/v_y ==
  Mode : Inport
  v_y_reset : Inport  Port=2
  reset : Inport  Port=3
  g(v) : Inport  Port=4
  f(v_n/V_R) : Inport  Port=5
  Gain : Gain  Gain=i_st_gy
  Initial Condition : InitialCondition  Value=0
  Integrator : Integrator  ExternalReset=either  InitialConditionSource=external  ShowStatePort=on
  Multiport Switch : MultiPortSwitch  Inputs=4
  Product : Product  RndMeth=Zero
  Sum2 : Sum  Inputs=++|
  alpha0 : Gain  Gain=alpha0_y
  alpha1 : Gain  Gain=alpha1_y
  alpha2 : Gain  Gain=alpha2_y
  alpha3 : Gain  Gain=alpha3_y
  v_y_out : Outport
  v_y_next : Outport  Port=2
  wires:
  Integrator/1 -> v_y_out/1, alpha1/1, alpha0/1, alpha2/1, alpha3/1  "v_y"
  alpha2/1 -> Multiport Switch/4
  Multiport Switch/1 -> Integrator/1
  Mode/1 -> Multiport Switch/1
  Integrator/State -> v_y_next/1
  reset/1 -> Integrator/2
  v_y_reset/1 -> Initial Condition/1
  Initial Condition/1 -> Integrator/3
  Gain/1 -> Sum2/1
  g(v)/1 -> Gain/1
  alpha0/1 -> Multiport Switch/2
  f(v_n/V_R)/1 -> Product/2
  alpha3/1 -> Product/1
  Product/1 -> Multiport Switch/5
  alpha1/1 -> Sum2/2
  Sum2/1 -> Multiport Switch/3

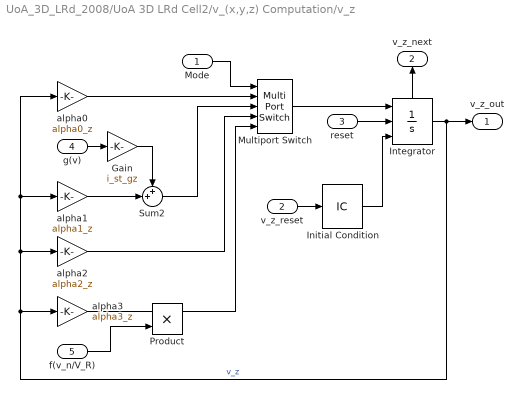
== system UoA_3D_LRd_2008/UoA 3D LRd Cell2/v_(x,y,z) Computation/v_z ==
  Mode : Inport
  v_z_reset : Inport  Port=2
  reset : Inport  Port=3
  g(v) : Inport  Port=4
  f(v_n/V_R) : Inport  Port=5
  Gain : Gain  Gain=i_st_gz
  Initial Condition : InitialCondition  Value=0
  Integrator : Integrator  ExternalReset=either  InitialConditionSource=external  ShowStatePort=on
  Multiport Switch : MultiPortSwitch  Inputs=4
  Product : Product  RndMeth=Zero
  Sum2 : Sum  Inputs=++|
  alpha0 : Gain  Gain=alpha0_z
  alpha1 : Gain  Gain=alpha1_z
  alpha2 : Gain  Gain=alpha2_z
  alpha3 : Gain  Gain=alpha3_z
  v_z_out : Outport
  v_z_next : Outport  Port=2
  wires:
  Integrator/1 -> v_z_out/1, alpha1/1, alpha0/1, alpha2/1, alpha3/1  "v_z"
  alpha2/1 -> Multiport Switch/4
  Multiport Switch/1 -> Integrator/1
  Mode/1 -> Multiport Switch/1
  Integrator/State -> v_z_next/1
  reset/1 -> Integrator/2
  v_z_reset/1 -> Initial Condition/1
  Initial Condition/1 -> Integrator/3
  g(v)/1 -> Gain/1
  Gain/1 -> Sum2/1
  alpha0/1 -> Multiport Switch/2
  alpha1/1 -> Sum2/2
  Sum2/1 -> Multiport Switch/3
  f(v_n/V_R)/1 -> Product/2
  alpha3/1 -> Multiport Switch/5

== system UoA_3D_LRd_2008/UoA 3D LRd Cell3/v_(x,y,z) Computation/f(v_n//V_R) ==
  v_n_R : Inport
  v_n_R_max : Inport  Port=2
  -10.99 : Gain  Gain=-10.99
  0.29 : Gain  Gain=0.29
  0.70 : Gain  Gain=0.70
  62.89 : Gain  Gain=62.89
  Subtract : Sum  Inputs=-+
  Sum3 : Sum  Inputs=|++
  Switch : Switch  Criteria=u2 > Threshold
  exp : Math  SaturateOnIntegerOverflow=on
  exp1 : Math  SaturateOnIntegerOverflow=on
  f(v_n/V_R) : Outport
  wires:
  Sum3/1 -> f(v_n/V_R)/1
  v_n_R_max/1 -> Switch/3, Subtract/2
  v_n_R/1 -> Switch/1, Subtract/1
  Subtract/1 -> Switch/2
  62.89/1 -> exp/1
  exp/1 -> 0.29/1
  -10.99/1 -> exp1/1
  exp1/1 -> 0.70/1
  0.29/1 -> Sum3/1
  0.70/1 -> Sum3/2
  Switch/1 -> 62.89/1, -10.99/1

== system UoA_3D_LRd_2008/UoA 3D LRd Cell3/v_(x,y,z) Computation/v_x ==
  Mode : Inport
  v_x_reset : Inport  Port=2
  reset : Inport  Port=3
  g(v) : Inport  Port=4
  f(v_n/V_R) : Inport  Port=5
  Gain : Gain  Gain=i_st_gx
  Initial Condition : InitialCondition  Value=0
  Integrator : Integrator  ExternalReset=either  InitialConditionSource=external  ShowStatePort=on
  Multiport Switch : MultiPortSwitch  Inputs=4
  Product : Product  RndMeth=Zero
  Sum1 : Sum  Inputs=++|
  alpha0 : Gain  Gain=alpha0_x
  alpha1 : Gain  Gain=alpha1_x
  alpha2 : Gain  Gain=alpha2_x
  alpha3 : Gain  Gain=alpha3_x
  v_x_out : Outport
  v_x_next : Outport  Port=2
  wires:
  alpha0/1 -> Multiport Switch/2
  alpha2/1 -> Multiport Switch/4
  Multiport Switch/1 -> Integrator/1
  Mode/1 -> Multiport Switch/1
  Gain/1 -> Sum1/1
  Integrator/1 -> alpha3/1, alpha1/1, alpha0/1, alpha2/1, v_x_out/1  "v_x"
  reset/1 -> Integrator/2
  v_x_reset/1 -> Initial Condition/1
  g(v)/1 -> Gain/1
  Initial Condition/1 -> Integrator/3
  Integrator/State -> v_x_next/1
  alpha1/1 -> Sum1/2
  Sum1/1 -> Multiport Switch/3
  f(v_n/V_R)/1 -> Product/2
  alpha3/1 -> Product/1
  Product/1 -> Multiport Switch/5

== system UoA_3D_LRd_2008/UoA 3D LRd Cell3/v_(x,y,z) Computation/v_y ==
  Mode : Inport
  v_y_reset : Inport  Port=2
  reset : Inport  Port=3
  g(v) : Inport  Port=4
  f(v_n/V_R) : Inport  Port=5
  Gain : Gain  Gain=i_st_gy
  Initial Condition : InitialCondition  Value=0
  Integrator : Integrator  ExternalReset=either  InitialConditionSource=external  ShowStatePort=on
  Multiport Switch : MultiPortSwitch  Inputs=4
  Product : Product  RndMeth=Zero
  Sum2 : Sum  Inputs=++|
  alpha0 : Gain  Gain=alpha0_y
  alpha1 : Gain  Gain=alpha1_y
  alpha2 : Gain  Gain=alpha2_y
  alpha3 : Gain  Gain=alpha3_y
  v_y_out : Outport
  v_y_next : Outport  Port=2
  wires:
  Integrator/1 -> v_y_out/1, alpha1/1, alpha0/1, alpha2/1, alpha3/1  "v_y"
  alpha2/1 -> Multiport Switch/4
  Multiport Switch/1 -> Integrator/1
  Mode/1 -> Multiport Switch/1
  Integrator/State -> v_y_next/1
  reset/1 -> Integrator/2
  v_y_reset/1 -> Initial Condition/1
  Initial Condition/1 -> Integrator/3
  Gain/1 -> Sum2/1
  g(v)/1 -> Gain/1
  alpha0/1 -> Multiport Switch/2
  f(v_n/V_R)/1 -> Product/2
  alpha3/1 -> Product/1
  Product/1 -> Multiport Switch/5
  alpha1/1 -> Sum2/2
  Sum2/1 -> Multiport Switch/3

== system UoA_3D_LRd_2008/UoA 3D LRd Cell3/v_(x,y,z) Computation/v_z ==
  Mode : Inport
  v_z_reset : Inport  Port=2
  reset : Inport  Port=3
  g(v) : Inport  Port=4
  Gain : Gain  Gain=i_st_gz
  Initial Condition : InitialCondition  Value=0
  Integrator : Integrator  ExternalReset=either  InitialConditionSource=external  ShowStatePort=on
  Multiport Switch : MultiPortSwitch  Inputs=4
  Sum2 : Sum  Inputs=++|
  alpha0 : Gain  Gain=alpha0_z
  alpha1 : Gain  Gain=alpha1_z
  alpha2 : Gain  Gain=alpha2_z
  alpha3 : Gain  Gain=alpha3_z
  v_z_out : Outport
  v_z_next : Outport  Port=2
  wires:
  Integrator/1 -> v_z_out/1, alpha1/1, alpha0/1, alpha2/1, alpha3/1  "v_z"
  alpha2/1 -> Multiport Switch/4
  Multiport Switch/1 -> Integrator/1
  Mode/1 -> Multiport Switch/1
  Integrator/State -> v_z_next/1
  reset/1 -> Integrator/2
  v_z_reset/1 -> Initial Condition/1
  Initial Condition/1 -> Integrator/3
  g(v)/1 -> Gain/1
  Gain/1 -> Sum2/1
  alpha0/1 -> Multiport Switch/2
  alpha1/1 -> Sum2/2
  Sum2/1 -> Multiport Switch/3
  alpha3/1 -> Multiport Switch/5

== system UoA_3D_LRd_2008/UoA 3D LRd Cell4/v_(x,y,z) Computation/f(v_n//V_R) ==
  v_n_R : Inport
  v_n_R_max : Inport  Port=2
  -10.99 : Gain  Gain=-10.99
  0.29 : Gain  Gain=0.29
  0.70 : Gain  Gain=0.70
  62.89 : Gain  Gain=62.89
  Subtract : Sum  Inputs=-+
  Sum3 : Sum  Inputs=|++
  Switch : Switch  Criteria=u2 > Threshold
  exp : Math  SaturateOnIntegerOverflow=on
  exp1 : Math  SaturateOnIntegerOverflow=on
  f(v_n/V_R) : Outport
  wires:
  Switch/1 -> -10.99/1, 62.89/1
  0.70/1 -> Sum3/2
  0.29/1 -> Sum3/1
  exp1/1 -> 0.70/1
  -10.99/1 -> exp1/1
  exp/1 -> 0.29/1
  62.89/1 -> exp/1
  Subtract/1 -> Switch/2
  v_n_R/1 -> Subtract/1, Switch/1
  v_n_R_max/1 -> Subtract/2, Switch/3
  Sum3/1 -> f(v_n/V_R)/1

== system UoA_3D_LRd_2008/UoA 3D LRd Cell4/v_(x,y,z) Computation/v_x ==
  Mode : Inport
  v_x_reset : Inport  Port=2
  reset : Inport  Port=3
  g(v) : Inport  Port=4
  f(v_n/V_R) : Inport  Port=5
  Gain : Gain  Gain=i_st_gx
  Initial Condition : InitialCondition  Value=0
  Integrator : Integrator  ExternalReset=either  InitialConditionSource=external  ShowStatePort=on
  Multiport Switch : MultiPortSwitch  DataPortOrder=Zero-based contiguous  Inputs=4
  Product : Product  RndMeth=Zero
  Sum1 : Sum  Inputs=++|
  alpha0 : Gain  Gain=alpha0_x
  alpha1 : Gain  Gain=alpha1_x
  alpha2 : Gain  Gain=alpha2_x
  alpha3 : Gain  Gain=alpha3_x
  v_x_out : Outport
  v_x_next : Outport  Port=2
  wires:
  Product/1 -> Multiport Switch/5
  alpha3/1 -> Product/1
  f(v_n/V_R)/1 -> Product/2
  Sum1/1 -> Multiport Switch/3
  alpha1/1 -> Sum1/2
  Integrator/State -> v_x_next/1
  Initial Condition/1 -> Integrator/3
  g(v)/1 -> Gain/1
  v_x_reset/1 -> Initial Condition/1
  reset/1 -> Integrator/2
  Integrator/1 -> v_x_out/1, alpha2/1, alpha0/1, alpha1/1, alpha3/1  "v_x"
  Gain/1 -> Sum1/1
  Mode/1 -> Multiport Switch/1
  Multiport Switch/1 -> Integrator/1
  alpha2/1 -> Multiport Switch/4
  alpha0/1 -> Multiport Switch/2

== system UoA_3D_LRd_2008/UoA 3D LRd Cell4/v_(x,y,z) Computation/v_y ==
  Mode : Inport
  v_y_reset : Inport  Port=2
  reset : Inport  Port=3
  g(v) : Inport  Port=4
  f(v_n/V_R) : Inport  Port=5
  Gain : Gain  Gain=i_st_gy
  Initial Condition : InitialCondition  Value=0
  Integrator : Integrator  ExternalReset=either  InitialConditionSource=external  ShowStatePort=on
  Multiport Switch : MultiPortSwitch  DataPortOrder=Zero-based contiguous  Inputs=4
  Product : Product  RndMeth=Zero
  Sum2 : Sum  Inputs=++|
  alpha0 : Gain  Gain=alpha0_y
  alpha1 : Gain  Gain=alpha1_y
  alpha2 : Gain  Gain=alpha2_y
  alpha3 : Gain  Gain=alpha3_y
  v_y_out : Outport
  v_y_next : Outport  Port=2
  wires:
  Sum2/1 -> Multiport Switch/3
  alpha1/1 -> Sum2/2
  Product/1 -> Multiport Switch/5
  alpha3/1 -> Product/1
  f(v_n/V_R)/1 -> Product/2
  alpha0/1 -> Multiport Switch/2
  g(v)/1 -> Gain/1
  Gain/1 -> Sum2/1
  Initial Condition/1 -> Integrator/3
  v_y_reset/1 -> Initial Condition/1
  reset/1 -> Integrator/2
  Integrator/State -> v_y_next/1
  Mode/1 -> Multiport Switch/1
  Multiport Switch/1 -> Integrator/1
  alpha2/1 -> Multiport Switch/4
  Integrator/1 -> alpha3/1, alpha2/1, alpha0/1, alpha1/1, v_y_out/1  "v_y"

== system UoA_3D_LRd_2008/UoA 3D LRd Cell4/v_(x,y,z) Computation/v_z ==
  Mode : Inport
  v_z_reset : Inport  Port=2
  reset : Inport  Port=3
  g(v) : Inport  Port=4
  Gain : Gain  Gain=i_st_gz
  Initial Condition : InitialCondition  Value=0
  Integrator : Integrator  ExternalReset=either  InitialConditionSource=external  ShowStatePort=on
  Multiport Switch : MultiPortSwitch  DataPortOrder=Zero-based contiguous  Inputs=4
  Sum2 : Sum  Inputs=++|
  alpha0 : Gain  Gain=alpha0_z
  alpha1 : Gain  Gain=alpha1_z
  alpha2 : Gain  Gain=alpha2_z
  alpha3 : Gain  Gain=alpha3_z
  v_z_out : Outport
  v_z_next : Outport  Port=2
  wires:
  alpha3/1 -> Multiport Switch/5
  Sum2/1 -> Multiport Switch/3
  alpha1/1 -> Sum2/2
  alpha0/1 -> Multiport Switch/2
  Gain/1 -> Sum2/1
  g(v)/1 -> Gain/1
  Initial Condition/1 -> Integrator/3
  v_z_reset/1 -> Initial Condition/1
  reset/1 -> Integrator/2
  Integrator/State -> v_z_next/1
  Mode/1 -> Multiport Switch/1
  Multiport Switch/1 -> Integrator/1
  alpha2/1 -> Multiport Switch/4
  Integrator/1 -> alpha3/1, alpha2/1, alpha0/1, alpha1/1, v_z_out/1  "v_z"

== stateflow chart UoA_3D_LRd_2008/UoA 3D LRd Cell1/Modes and Transitions ==
  settings: sampleTime=inf  executeAtInitialization=1
  state Resting_FR
    entry: Mode = 1;
  state Stimulated
    entry: Mode = 2;
  state Upstroke
    entry: Mode = 3;
  state Plateau_ER
    entry: Mode = 4;
  (default) -> Resting_FR
  Resting_FR -> Stimulated : [(stimulus > 0) && ((v_x - v_y + v_z) <= V_T)] /
      | v_x_reset = v_x;
      | v_y_reset = v_y;
      | v_z_reset = v_z;
      | v_n_R = (v_x - v_y + v_z)/V_R;
      | V_O = V_O_max - 80.1*sqrt((v_x - v_y + v_z)/V_R);
      | reset;
  Stimulated -> Resting_FR [order 2] : [(stimulus <= 0) && ((v_x - v_y + v_z) < V_T)] /
      | v_x_reset = v_x;
      | v_y_reset = v_y;
      | v_z_reset = v_z;
      | reset;
  Plateau_ER -> Resting_FR : [(v_x - v_y + v_z) <= V_R] /
      | v_x_reset = v_x;
      | v_y_reset = v_y;
      | v_z_reset = v_z;
      | reset;
  Stimulated -> Upstroke [order 1] : [(v_x - v_y + v_z) >= V_T] /
      | v_x_reset = v_x;
      | v_y_reset = v_y;
      | v_z_reset = v_z;
      | reset;
  Upstroke -> Plateau_ER : [(v_x - v_y + v_z) >= V_O] /
      | v_x_reset = v_x;
      | v_y_reset = v_y;
      | v_z_reset = v_z;
      | reset;
  data: stimulus input double; V_T input double; V_R input double; V_O_max input double; v_x input double size=1; v_y input double size=1; v_z input double size=1; Mode output double size=1 [1..4] =1; v_n_R output double =0; v_x_reset output double =0; v_y_reset output double =0; v_z_reset output double =0; V_O local double
  events: reset output EITHER_EDGE_EVENT

== stateflow chart UoA_3D_LRd_2008/UoA 3D LRd Cell2/Modes and Transitions ==
  settings: sampleTime=inf  executeAtInitialization=1
  state Resting_FR
    entry: Mode = 1;
  state Stimulated
    entry: Mode = 2;
  state Upstroke
    entry: Mode = 3;
  state Plateau_ER
    entry: Mode = 4;
  (default) -> Resting_FR
  Resting_FR -> Stimulated : [(stimulus > V_T) && ((v_x - v_y + v_z) <= V_T)] /
      | v_x_reset = v_x;
      | v_y_reset = v_y;
      | v_z_reset = v_z;
      | v_n_R = (v_x - v_y + v_z)/V_R;
      | V_O = V_O_max - 80.1*sqrt((v_x - v_y + v_z)/V_R);
      | reset;
  Stimulated -> Resting_FR [order 2] : [(stimulus <= 0) && ((v_x - v_y + v_z) < V_T)] /
      | v_x_reset = v_x;
      | v_y_reset = v_y;
      | v_z_reset = v_z;
      | reset;
  Plateau_ER -> Resting_FR : [(v_x - v_y + v_z) <= V_R] /
      | v_x_reset = v_x;
      | v_y_reset = v_y;
      | v_z_reset = v_z;
      | reset;
  Stimulated -> Upstroke [order 1] : [(v_x - v_y + v_z) >= V_T] /
      | v_x_reset = v_x;
      | v_y_reset = v_y;
      | v_z_reset = v_z;
      | reset;
  Upstroke -> Plateau_ER : [(v_x - v_y + v_z) >= V_O] /
      | v_x_reset = v_x;
      | v_y_reset = v_y;
      | v_z_reset = v_z;
      | reset;
  data: stimulus input double; V_T input double; V_R input double; V_O_max input double; v_x input double size=1; v_y input double size=1; v_z input double size=1; Mode output double size=1 [1..4] =1; v_n_R output double =0; v_x_reset output double =0; v_y_reset output double =0; v_z_reset output double =0; V_O local double
  events: reset output EITHER_EDGE_EVENT

== stateflow chart UoA_3D_LRd_2008/UoA 3D LRd Cell3/Modes and Transitions ==
  settings: sampleTime=inf  executeAtInitialization=1
  state Resting_FR
    entry: Mode = 1;
  state Stimulated
    entry: Mode = 2;
  state Upstroke
    entry: Mode = 3;
  state Plateau_ER
    entry: Mode = 4;
  (default) -> Resting_FR
  Resting_FR -> Stimulated : [(stimulus > V_T) && ((v_x - v_y + v_z) <= V_T)] /
      | v_x_reset = v_x;
      | v_y_reset = v_y;
      | v_z_reset = v_z;
      | v_n_R = (v_x - v_y + v_z)/V_R;
      | V_O = V_O_max - 80.1*sqrt((v_x - v_y + v_z)/V_R);
      | reset;
  Stimulated -> Resting_FR [order 2] : [(stimulus <= 0) && ((v_x - v_y + v_z) < V_T)] /
      | v_x_reset = v_x;
      | v_y_reset = v_y;
      | v_z_reset = v_z;
      | reset;
  Plateau_ER -> Resting_FR : [(v_x - v_y + v_z) <= V_R] /
      | v_x_reset = v_x;
      | v_y_reset = v_y;
      | v_z_reset = v_z;
      | reset;
  Stimulated -> Upstroke [order 1] : [(v_x - v_y + v_z) >= V_T] /
      | v_x_reset = v_x;
      | v_y_reset = v_y;
      | v_z_reset = v_z;
      | reset;
  Upstroke -> Plateau_ER : [(v_x - v_y + v_z) >= V_O] /
      | v_x_reset = v_x;
      | v_y_reset = v_y;
      | v_z_reset = v_z;
      | reset;
  data: stimulus input double; V_T input double; V_R input double; V_O_max input double; v_x input double size=1; v_y input double size=1; v_z input double size=1; Mode output double size=1 [1..4] =1; v_n_R output double =0; v_x_reset output double =0; v_y_reset output double =0; v_z_reset output double =0; V_O local double
  events: reset output EITHER_EDGE_EVENT

== stateflow chart UoA_3D_LRd_2008/UoA Path 1/Modes and Transitions ==
  settings: updateMethod=CONTINUOUS  executeAtInitialization=1
  state Replay_cell1
  state Replay_cell2
  state Previous_Direction1
  state Idle
  state Previous_Direction2
  state Wait_cell2
  state Wait_cell1
  state Annihilate
  Wait_cell1 -> Replay_cell1 [order 2] : after(cell1_conduction_time, sec) /
      | cell1_replay = 1;
      | from_cell = 1;
  Wait_cell2 -> Replay_cell2 [order 2] : after(cell2_conduction_time, sec) /
      | cell2_replay = 1;
      | from_cell = 2;
  Replay_cell1 -> Idle : after(cell2_charge_time, sec) /
      | cell1_replay = 0;
  Replay_cell2 -> Idle : after(cell1_charge_time, sec) /
      | cell2_replay = 0;
  (default) -> Idle
  Idle -> Previous_Direction2 [order 3] : [cell2_mode == 2 ...
      | && cell1_mode != 2]
  Previous_Direction2 -> Wait_cell2 [order 2] : [from_cell == 0]
  Idle -> Previous_Direction1 [order 2] : [cell1_mode == 2 ...
      | && cell2_mode != 2]
  Previous_Direction1 -> Wait_cell1 [order 2] : [from_cell == 0]
  Idle -> Annihilate [order 1] : [cell1_mode == 2 ...
      | && cell2_mode == 2]
  Annihilate -> Idle : [cell1_mode != 2 ...
      | && cell2_mode != 2] /
      | from_cell = 0;
  Previous_Direction2 -> Wait_cell2 [order 3] : [from_cell == 2]
  Previous_Direction1 -> Wait_cell1 [order 3] : [from_cell == 1]
  Previous_Direction2 -> Wait_cell2 [order 4] : [from_cell == 1 && ...
      | cell1_mode_delayed == 0]
  Previous_Direction1 -> Wait_cell1 [order 4] : [from_cell == 2 && ...
      | cell2_mode_delayed == 0]
  Wait_cell2 -> Annihilate [order 1] : [cell1_mode == 2]
  Wait_cell1 -> Annihilate [order 1] : [cell2_mode == 2]
  Previous_Direction1 -> Annihilate [order 1] : [from_cell == 2 && ...
      | cell2_mode_delayed != 0]
  Previous_Direction2 -> Annihilate [order 1] : [from_cell == 1 && ...
      | cell1_mode_delayed != 0]
  data: cell1_mode input double; cell1_conduction_time parameter double; cell1_mode_delayed input double; cell2_mode input double; cell2_conduction_time parameter double; cell1_replay output boolean =0; cell2_replay output boolean =0; cell2_mode_delayed input double; cell1_charge_time parameter double; cell2_charge_time parameter double; from_cell local int8 [0..2] =0

== stateflow chart UoA_3D_LRd_2008/UoA 3D LRd Cell4/Modes and Transitions ==
  settings: sampleTime=inf  executeAtInitialization=1
  state Resting_FR
    entry: Mode = 0;
  state Stimulated
    entry: Mode = 1;
  state Upstroke
    entry: Mode = 2;
  state Plateau_ER
    entry: Mode = 3;
  (default) -> Resting_FR
  Resting_FR -> Stimulated : [(stimulus > V_T) && ((v_x - v_y + v_z) <= V_T)] /
      | v_x_reset = (v_x - v_y + v_z)*0.3;
      | v_y_reset = (v_x - v_y + v_z)*0.0;
      | v_z_reset = (v_x - v_y + v_z)*0.7;
      | v_n_R = (v_x - v_y + v_z)/V_R;
      | V_O = V_O_max - 80.1*sqrt((v_x - v_y + v_z)/V_R);
      | reset;
  Stimulated -> Resting_FR [order 2] : [(stimulus <= 0) && ((v_x - v_y + v_z) < V_T)] /
      | v_x_reset = v_x;
      | v_y_reset = v_y;
      | v_z_reset = v_z;
      | reset;
  Plateau_ER -> Resting_FR : [(v_x - v_y + v_z) <= V_R] /
      | v_x_reset = v_x;
      | v_y_reset = v_y;
      | v_z_reset = v_z;
      | reset;
  Stimulated -> Upstroke [order 1] : [(v_x - v_y + v_z) >= V_T] /
      | v_x_reset = v_x;
      | v_y_reset = v_y;
      | v_z_reset = v_z;
      | reset;
  Upstroke -> Plateau_ER : [(v_x - v_y + v_z) >= V_O] /
      | v_x_reset = v_x;
      | v_y_reset = v_y;
      | v_z_reset = v_z;
      | reset;
  data: stimulus input double; V_T input double; V_R input double; V_O_max input double; v_x input double size=1; v_y input double size=1; v_z input double size=1; Mode output double size=1 [0..3] =0; v_n_R output double =0; v_x_reset output double =0; v_y_reset output double =0; v_z_reset output double =0; V_O local double
  events: reset output EITHER_EDGE_EVENT
